simulink model "case1"  (R2024b)
settings: Solver=FixedStepAuto  StartTime=0  StopTime=1  FixedStep=1e-7  RelTol=1e-3
values from neighbouring files (symbols this model uses):
  SG_D_1_D = 0.01056    [IEEE9_case_parameters.m]    (also in case1_parameters.m; case2_parameters.m; case3_parameters.m; case4_parameters.m)
  SG_D_1_EnableSaturation = 0    [IEEE9_case_parameters.m]    (also in case1_parameters.m; case2_parameters.m; case3_parameters.m; case4_parameters.m)
  SG_D_1_f0 = 60    [IEEE9_case_parameters.m]    (also in case1_parameters.m; case2_parameters.m; case3_parameters.m; case4_parameters.m)
  SG_D_1_H = 7.5    [IEEE9_case_parameters.m]    (also in case1_parameters.m; case2_parameters.m; case3_parameters.m; case4_parameters.m)
  SG_D_1_K_A = 20    [IEEE9_case_parameters.m]    (also in case1_parameters.m; case2_parameters.m; case3_parameters.m; case4_parameters.m)
  SG_D_1_K_E = 1.000000e+1    (= 10)    [IEEE9_case_parameters.m]    (also in case1_parameters.m; case2_parameters.m; case3_parameters.m; case4_parameters.m)
  SG_D_1_K_F = 2.363    [IEEE9_case_parameters.m]    (also in case1_parameters.m; case2_parameters.m; case3_parameters.m; case4_parameters.m)
  SG_D_1_K_s = 0.5    [IEEE9_case_parameters.m]    (also in case1_parameters.m = 5; case2_parameters.m = 5; case3_parameters.m = 5; case4_parameters.m = 5)
  SG_D_1_R_a = 0.001088    [IEEE9_case_parameters.m]    (also in case1_parameters.m; case2_parameters.m; case3_parameters.m; case4_parameters.m)
  SG_D_1_S_A = 1    [IEEE9_case_parameters.m]    (also in case1_parameters.m; case2_parameters.m; case3_parameters.m; case4_parameters.m)
  SG_D_1_S_B = 0.103    [IEEE9_case_parameters.m]    (also in case1_parameters.m; case2_parameters.m; case3_parameters.m; case4_parameters.m)
  SG_D_1_S_N = 10.659857    [IEEE9_case_parameters.m]    (also in case1_parameters.m; case2_parameters.m; case3_parameters.m; case4_parameters.m)
  SG_D_1_SpeedPara = 200    [IEEE9_case_parameters.m]    (also in case1_parameters.m; case2_parameters.m; case3_parameters.m; case4_parameters.m)
  SG_D_1_T_0 = 0.720173    [IEEE9_case_parameters.m]    (also in case1_parameters.m = 0.755522; case2_parameters.m = 0.808931; case3_parameters.m = 0.869402; case4_parameters.m = 0.729316)
  SG_D_1_T_1 = 0.3    [IEEE9_case_parameters.m]    (also in case1_parameters.m; case2_parameters.m; case3_parameters.m; case4_parameters.m)
  SG_D_1_T_2 = 0.05    [IEEE9_case_parameters.m]    (also in case1_parameters.m; case2_parameters.m; case3_parameters.m; case4_parameters.m)
  SG_D_1_T_3 = 0.02    [IEEE9_case_parameters.m]    (also in case1_parameters.m; case2_parameters.m; case3_parameters.m; case4_parameters.m)
  SG_D_1_T_4 = 0.005    [IEEE9_case_parameters.m]    (also in case1_parameters.m; case2_parameters.m; case3_parameters.m; case4_parameters.m)
  SG_D_1_T_A = 0.02    [IEEE9_case_parameters.m]    (also in case1_parameters.m; case2_parameters.m; case3_parameters.m; case4_parameters.m)
  SG_D_1_T_dd = 8.000000e+0    (= 8)    [IEEE9_case_parameters.m]    (also in case1_parameters.m; case2_parameters.m; case3_parameters.m; case4_parameters.m)
  SG_D_1_T_ddd = 0.04    [IEEE9_case_parameters.m]    (also in case1_parameters.m; case2_parameters.m; case3_parameters.m; case4_parameters.m)
  SG_D_1_T_E = 0.314    [IEEE9_case_parameters.m]    (also in case1_parameters.m; case2_parameters.m; case3_parameters.m; case4_parameters.m)
  SG_D_1_T_F = 0.35    [IEEE9_case_parameters.m]    (also in case1_parameters.m; case2_parameters.m; case3_parameters.m; case4_parameters.m)
  SG_D_1_T_qd = 0.8    [IEEE9_case_parameters.m]    (also in case1_parameters.m; case2_parameters.m; case3_parameters.m; case4_parameters.m)
  SG_D_1_T_qdd = 0.02    [IEEE9_case_parameters.m]    (also in case1_parameters.m; case2_parameters.m; case3_parameters.m; case4_parameters.m)
  SG_D_1_T_speed = 0.1    [IEEE9_case_parameters.m]    (also in case1_parameters.m = 200; case2_parameters.m = 200; case3_parameters.m = 200; case4_parameters.m = 200)
  SG_D_1_T_w = 0.5    [IEEE9_case_parameters.m]    (also in case1_parameters.m; case2_parameters.m; case3_parameters.m; case4_parameters.m)
  SG_D_1_V_ref = 1.990276    [IEEE9_case_parameters.m]    (also in case1_parameters.m = 2.042296; case2_parameters.m = 2.051388; case3_parameters.m = 2.089584; case4_parameters.m = 2.01845)
  SG_D_1_w_ref = 376.991118    [IEEE9_case_parameters.m]    (also in case1_parameters.m; case2_parameters.m; case3_parameters.m; case4_parameters.m)
  SG_D_1_wb = 6.000000e+1    (= 60)    [IEEE9_case_parameters.m]    (also in case1_parameters.m; case2_parameters.m; case3_parameters.m; case4_parameters.m)
  SG_D_1_x_d = 1.9    [IEEE9_case_parameters.m]    (also in case1_parameters.m; case2_parameters.m; case3_parameters.m; case4_parameters.m)
  SG_D_1_x_dd = 0.302    [IEEE9_case_parameters.m]    (also in case1_parameters.m; case2_parameters.m; case3_parameters.m; case4_parameters.m)
  SG_D_1_x_ddd = 0.204    [IEEE9_case_parameters.m]    (also in case1_parameters.m; case2_parameters.m; case3_parameters.m; case4_parameters.m)
  SG_D_1_x_l = 0.05    [IEEE9_case_parameters.m]    (also in case1_parameters.m; case2_parameters.m; case3_parameters.m; case4_parameters.m)
  SG_D_1_x_q = 1.3    [IEEE9_case_parameters.m]    (also in case1_parameters.m; case2_parameters.m; case3_parameters.m; case4_parameters.m)
  SG_D_1_x_qd = 0.5    [IEEE9_case_parameters.m]    (also in case1_parameters.m; case2_parameters.m; case3_parameters.m; case4_parameters.m)
  SG_D_1_x_qdd = 0.3    [IEEE9_case_parameters.m]    (also in case1_parameters.m; case2_parameters.m; case3_parameters.m; case4_parameters.m)
  SG_D_2_D = 0.02    [IEEE9_case_parameters.m]    (also in case1_parameters.m; case2_parameters.m; case3_parameters.m; case4_parameters.m)
  SG_D_2_EnableSaturation = 0    [IEEE9_case_parameters.m]    (also in case1_parameters.m; case2_parameters.m; case3_parameters.m; case4_parameters.m)
  SG_D_2_f0 = 60    [IEEE9_case_parameters.m]    (also in case1_parameters.m; case2_parameters.m; case3_parameters.m; case4_parameters.m)
  SG_D_2_H = 8.000000e+0    (= 8)    [IEEE9_case_parameters.m]    (also in case1_parameters.m; case2_parameters.m; case3_parameters.m; case4_parameters.m)
  SG_D_2_K_A = 20    [IEEE9_case_parameters.m]    (also in case1_parameters.m; case2_parameters.m; case3_parameters.m; case4_parameters.m)
  SG_D_2_K_E = 1.000000e+1    (= 10)    [IEEE9_case_parameters.m]    (also in case1_parameters.m; case2_parameters.m; case3_parameters.m; case4_parameters.m)
  SG_D_2_K_F = 2.363    [IEEE9_case_parameters.m]    (also in case1_parameters.m; case2_parameters.m; case3_parameters.m; case4_parameters.m)
  SG_D_2_K_s = 0.5    [IEEE9_case_parameters.m]    (also in case1_parameters.m = 4; case2_parameters.m = 4; case3_parameters.m = 4; case4_parameters.m = 4)
  SG_D_2_R_a = 0.001088    [IEEE9_case_parameters.m]    (also in case1_parameters.m; case2_parameters.m; case3_parameters.m; case4_parameters.m)
  SG_D_2_S_A = 1    [IEEE9_case_parameters.m]    (also in case1_parameters.m; case2_parameters.m; case3_parameters.m; case4_parameters.m)
  SG_D_2_S_B = 0.103    [IEEE9_case_parameters.m]    (also in case1_parameters.m; case2_parameters.m; case3_parameters.m; case4_parameters.m)
  SG_D_2_S_N = 10.659857    [IEEE9_case_parameters.m]    (also in case1_parameters.m; case2_parameters.m; case3_parameters.m; case4_parameters.m)
  SG_D_2_SpeedPara = 200    [IEEE9_case_parameters.m]    (also in case1_parameters.m; case2_parameters.m; case3_parameters.m; case4_parameters.m)
  SG_D_2_T_0 = 1.632913    [IEEE9_case_parameters.m]    (also in case1_parameters.m = 1.632925; case2_parameters.m = 1.632915; case3_parameters.m = 1.632914; case4_parameters.m = 1.632927)
  SG_D_2_T_1 = 0.2    [IEEE9_case_parameters.m]    (also in case1_parameters.m; case2_parameters.m; case3_parameters.m; case4_parameters.m)
  SG_D_2_T_2 = 0.05    [IEEE9_case_parameters.m]    (also in case1_parameters.m; case2_parameters.m; case3_parameters.m; case4_parameters.m)
  SG_D_2_T_3 = 0.02    [IEEE9_case_parameters.m]    (also in case1_parameters.m; case2_parameters.m; case3_parameters.m; case4_parameters.m)
  SG_D_2_T_4 = 0.005    [IEEE9_case_parameters.m]    (also in case1_parameters.m; case2_parameters.m; case3_parameters.m; case4_parameters.m)
  SG_D_2_T_A = 0.02    [IEEE9_case_parameters.m]    (also in case1_parameters.m; case2_parameters.m; case3_parameters.m; case4_parameters.m)
  SG_D_2_T_dd = 7.9    [IEEE9_case_parameters.m]    (also in case1_parameters.m; case2_parameters.m; case3_parameters.m; case4_parameters.m)
  SG_D_2_T_ddd = 0.04    [IEEE9_case_parameters.m]    (also in case1_parameters.m; case2_parameters.m; case3_parameters.m; case4_parameters.m)
  SG_D_2_T_E = 0.314    [IEEE9_case_parameters.m]    (also in case1_parameters.m; case2_parameters.m; case3_parameters.m; case4_parameters.m)
  SG_D_2_T_F = 0.35    [IEEE9_case_parameters.m]    (also in case1_parameters.m; case2_parameters.m; case3_parameters.m; case4_parameters.m)
  SG_D_2_T_qd = 0.8    [IEEE9_case_parameters.m]    (also in case1_parameters.m; case2_parameters.m; case3_parameters.m; case4_parameters.m)
  SG_D_2_T_qdd = 0.015    [IEEE9_case_parameters.m]    (also in case1_parameters.m; case2_parameters.m; case3_parameters.m; case4_parameters.m)
  SG_D_2_T_speed = 0.1    [IEEE9_case_parameters.m]    (also in case1_parameters.m = 150; case2_parameters.m = 150; case3_parameters.m = 150; case4_parameters.m = 150)
  SG_D_2_T_w = 0.35    [IEEE9_case_parameters.m]    (also in case1_parameters.m; case2_parameters.m; case3_parameters.m; case4_parameters.m)
  SG_D_2_V_ref = 2.58547    [IEEE9_case_parameters.m]    (also in case1_parameters.m = 2.597896; case2_parameters.m = 2.587136; case3_parameters.m = 2.586042; case4_parameters.m = 2.599679)
  SG_D_2_w_ref = 376.991118    [IEEE9_case_parameters.m]    (also in case1_parameters.m; case2_parameters.m; case3_parameters.m; case4_parameters.m)
  SG_D_2_wb = 6.000000e+1    (= 60)    [IEEE9_case_parameters.m]    (also in case1_parameters.m; case2_parameters.m; case3_parameters.m; case4_parameters.m)
  SG_D_2_x_d = 1.8    [IEEE9_case_parameters.m]    (also in case1_parameters.m; case2_parameters.m; case3_parameters.m; case4_parameters.m)
  SG_D_2_x_dd = 0.302    [IEEE9_case_parameters.m]    (also in case1_parameters.m; case2_parameters.m; case3_parameters.m; case4_parameters.m)
  SG_D_2_x_ddd = 0.204    [IEEE9_case_parameters.m]    (also in case1_parameters.m; case2_parameters.m; case3_parameters.m; case4_parameters.m)
  SG_D_2_x_l = 0.05    [IEEE9_case_parameters.m]    (also in case1_parameters.m; case2_parameters.m; case3_parameters.m; case4_parameters.m)
  SG_D_2_x_q = 1.25    [IEEE9_case_parameters.m]    (also in case1_parameters.m; case2_parameters.m; case3_parameters.m; case4_parameters.m)
  SG_D_2_x_qd = 0.5    [IEEE9_case_parameters.m]    (also in case1_parameters.m; case2_parameters.m; case3_parameters.m; case4_parameters.m)
  SG_D_2_x_qdd = 0.3    [IEEE9_case_parameters.m]    (also in case1_parameters.m; case2_parameters.m; case3_parameters.m; case4_parameters.m)
  SG_D_3_D = 0.02    [IEEE9_case_parameters.m]    (also in case1_parameters.m; case2_parameters.m; case3_parameters.m; case4_parameters.m)
  SG_D_3_EnableSaturation = 0    [IEEE9_case_parameters.m]    (also in case1_parameters.m; case2_parameters.m; case3_parameters.m; case4_parameters.m)
  SG_D_3_f0 = 60    [IEEE9_case_parameters.m]    (also in case1_parameters.m; case2_parameters.m; case3_parameters.m; case4_parameters.m)
  SG_D_3_H = 7.7    [IEEE9_case_parameters.m]    (also in case1_parameters.m; case2_parameters.m; case3_parameters.m; case4_parameters.m)
  SG_D_3_K_A = 20    [IEEE9_case_parameters.m]    (also in case1_parameters.m; case2_parameters.m; case3_parameters.m; case4_parameters.m)
  SG_D_3_K_E = 1.000000e+1    (= 10)    [IEEE9_case_parameters.m]    (also in case1_parameters.m; case2_parameters.m; case3_parameters.m; case4_parameters.m)
  SG_D_3_K_F = 2.363    [IEEE9_case_parameters.m]    (also in case1_parameters.m; case2_parameters.m; case3_parameters.m; case4_parameters.m)
  SG_D_3_K_s = 0.2    [IEEE9_case_parameters.m]    (also in case1_parameters.m = 2; case2_parameters.m = 2; case3_parameters.m = 2; case4_parameters.m = 2)
  SG_D_3_R_a = 0.001088    [IEEE9_case_parameters.m]    (also in case1_parameters.m; case2_parameters.m; case3_parameters.m; case4_parameters.m)
  SG_D_3_S_A = 1    [IEEE9_case_parameters.m]    (also in case1_parameters.m; case2_parameters.m; case3_parameters.m; case4_parameters.m)
  SG_D_3_S_B = 0.103    [IEEE9_case_parameters.m]    (also in case1_parameters.m; case2_parameters.m; case3_parameters.m; case4_parameters.m)
  SG_D_3_S_N = 10.659857    [IEEE9_case_parameters.m]    (also in case1_parameters.m; case2_parameters.m; case3_parameters.m; case4_parameters.m)
  SG_D_3_SpeedPara = 200    [IEEE9_case_parameters.m]    (also in case1_parameters.m; case2_parameters.m; case3_parameters.m; case4_parameters.m)
  SG_D_3_T_0 = 0.850788    [IEEE9_case_parameters.m]    (also in case1_parameters.m = 0.850786; case2_parameters.m = 0.850787; case3_parameters.m; case4_parameters.m = 0.850786)
  SG_D_3_T_1 = 0.2    [IEEE9_case_parameters.m]    (also in case1_parameters.m; case2_parameters.m; case3_parameters.m; case4_parameters.m)
  SG_D_3_T_2 = 0.05    [IEEE9_case_parameters.m]    (also in case1_parameters.m; case2_parameters.m; case3_parameters.m; case4_parameters.m)
  SG_D_3_T_3 = 0.02    [IEEE9_case_parameters.m]    (also in case1_parameters.m; case2_parameters.m; case3_parameters.m; case4_parameters.m)
  SG_D_3_T_4 = 0.005    [IEEE9_case_parameters.m]    (also in case1_parameters.m; case2_parameters.m; case3_parameters.m; case4_parameters.m)
  SG_D_3_T_A = 0.02    [IEEE9_case_parameters.m]    (also in case1_parameters.m; case2_parameters.m; case3_parameters.m; case4_parameters.m)
  SG_D_3_T_dd = 8.1    [IEEE9_case_parameters.m]    (also in case1_parameters.m; case2_parameters.m; case3_parameters.m; case4_parameters.m)
  SG_D_3_T_ddd = 0.04    [IEEE9_case_parameters.m]    (also in case1_parameters.m; case2_parameters.m; case3_parameters.m; case4_parameters.m)
  SG_D_3_T_E = 0.314    [IEEE9_case_parameters.m]    (also in case1_parameters.m; case2_parameters.m; case3_parameters.m; case4_parameters.m)
  SG_D_3_T_F = 0.35    [IEEE9_case_parameters.m]    (also in case1_parameters.m; case2_parameters.m; case3_parameters.m; case4_parameters.m)
  SG_D_3_T_qd = 0.8    [IEEE9_case_parameters.m]    (also in case1_parameters.m; case2_parameters.m; case3_parameters.m; case4_parameters.m)
  SG_D_3_T_qdd = 0.015    [IEEE9_case_parameters.m]    (also in case1_parameters.m; case2_parameters.m; case3_parameters.m; case4_parameters.m)
  SG_D_3_T_speed = 0.1    [IEEE9_case_parameters.m]    (also in case1_parameters.m = 180; case2_parameters.m = 180; case3_parameters.m = 180; case4_parameters.m = 180)
  SG_D_3_T_w = 0.4    [IEEE9_case_parameters.m]    (also in case1_parameters.m; case2_parameters.m; case3_parameters.m; case4_parameters.m)
  SG_D_3_V_ref = 1.892727    [IEEE9_case_parameters.m]    (also in case1_parameters.m = 1.906439; case2_parameters.m = 1.895535; case3_parameters.m = 1.892105; case4_parameters.m = 1.906598)
  SG_D_3_w_ref = 376.991118    [IEEE9_case_parameters.m]    (also in case1_parameters.m; case2_parameters.m; case3_parameters.m; case4_parameters.m)
  SG_D_3_wb = 6.000000e+1    (= 60)    [IEEE9_case_parameters.m]    (also in case1_parameters.m; case2_parameters.m; case3_parameters.m; case4_parameters.m)
  SG_D_3_x_d = 1.85    [IEEE9_case_parameters.m]    (also in case1_parameters.m; case2_parameters.m; case3_parameters.m; case4_parameters.m)
  SG_D_3_x_dd = 0.302    [IEEE9_case_parameters.m]    (also in case1_parameters.m; case2_parameters.m; case3_parameters.m; case4_parameters.m)
  SG_D_3_x_ddd = 0.204    [IEEE9_case_parameters.m]    (also in case1_parameters.m; case2_parameters.m; case3_parameters.m; case4_parameters.m)
  SG_D_3_x_l = 0.05    [IEEE9_case_parameters.m]    (also in case1_parameters.m; case2_parameters.m; case3_parameters.m; case4_parameters.m)
  SG_D_3_x_q = 1.2    [IEEE9_case_parameters.m]    (also in case1_parameters.m; case2_parameters.m; case3_parameters.m; case4_parameters.m)
  SG_D_3_x_qd = 0.5    [IEEE9_case_parameters.m]    (also in case1_parameters.m; case2_parameters.m; case3_parameters.m; case4_parameters.m)
  SG_D_3_x_qdd = 0.3    [IEEE9_case_parameters.m]    (also in case1_parameters.m; case2_parameters.m; case3_parameters.m; case4_parameters.m)
(part 8 of 12)

== system case1/SG_D_2/d_psi_d_SG_D_2_block ==
  note: d_psi_d_SG_D_2 in case1
      | $2\,\pi \,f_{0}\,\left(v_{d,\mathrm{SG},D,2}\,\sin\left(\theta _{\mathrm{SG},D,2}\right)-v_{q,\mathrm{SG},D,2}\,\cos\left(\theta _{\mathrm{SG},D,2}\right)+\frac{R_{a}\,\left(\frac{\psi _{\mathrm{1d},\mathrm{SG},D,2}\,\left(x_{\mathrm{dd}}-x_{\mathrm{ddd}}\right)}{x_{\mathrm{dd}}-x_{l}}-\psi _{d,\mathrm{SG},D,2}+\frac{\psi _{\mathrm{fd},\mathrm{SG},D,2}\,\left(x_{\mathrm{ddd}}-x_{l}\right)}{x_{\mathrm{dd}}-x_{l}}\right)}{x_{\mathrm{ddd}}}+\frac{\psi _{q,\mathrm{SG},D,2}\,w_{\mathrm{SG},D,2}}{2\,f_{0}\,\pi }\right)$
      | Automatically generated on 2025-10-31 18:48:10 .
  State_psi_1d_SG_D_2_48ea4 : Inport
  State_psi_d_SG_D_2_8d25d : Inport  Port=2
  State_psi_fd_SG_D_2_4d493 : Inport  Port=3
  Input_v_d_SG_D_2_e74d4 : Inport  Port=4
  State_theta_SG_D_2_cb884 : Inport  Port=5
  Input_v_q_SG_D_2_ef7b1 : Inport  Port=6
  State_theta_SG_D_2_069cc : Inport  Port=7
  State_psi_q_SG_D_2_06491 : Inport  Port=8
  State_w_SG_D_2_46e5d : Inport  Port=9
  Add_9594a : Sum
  Add_a58f5 : Sum
  Constant_-1_bbc80 : Constant  Value=-1
  Constant_-2.0_5abee : Constant  Value=-2.0
  Constant_2.0_c2643 : Constant  Value=2.0
  Constant_R_a_77be8 : Constant  Value=R_a
  Constant_f0_ecad6 : Constant  Value=f0
  Constant_f0_ecc70 : Constant  Value=f0
  Constant_pi_1b2b5 : Constant  Value=pi
  Constant_pi_ab6a4 : Constant  Value=pi
  Constant_x_dd_4634c : Constant  Value=x_dd
  Constant_x_dd_53177 : Constant  Value=x_dd
  Constant_x_dd_7f193 : Constant  Value=x_dd
  Constant_x_ddd_27663 : Constant  Value=x_ddd
  Constant_x_ddd_2f050 : Constant  Value=x_ddd
  Constant_x_ddd_407bb : Constant  Value=x_ddd
  Constant_x_l_0d10b : Constant  Value=x_l
  Constant_x_l_b133c : Constant  Value=x_l
  Constant_x_l_d501e : Constant  Value=x_l
  Divide_2553b : Product  Inputs=*/
  Divide_6fe8b : Product  Inputs=*/
  Divide_88a68 : Product  Inputs=*/
  Divide_89ce0 : Product  Inputs=*/
  MathFunc_cos_0fde2 : Trigonometry  Operator=cos
  MathFunc_sin_788f3 : Trigonometry
  Product_269c7 : Product
  Product_5eb09 : Product
  Product_94f92 : Product
  Product_9e7bd : Product
  Product_a0a07 : Product
  Product_b26e1 : Product
  Product_d5dea : Product
  Product_d6782 : Product
  Product_ea208 : Product
  Product_eca76 : Product
  Product_f9e18 : Product
  Product_fe3b7 : Product
  Subtract_6ad03 : Sum  Inputs=+-
  Subtract_6defb : Sum  Inputs=+-
  Subtract_826d9 : Sum  Inputs=+-
  Subtract_837ee : Sum  Inputs=+-
  Subtract_881d5 : Sum  Inputs=+-
  Subtract_8d79c : Sum  Inputs=+-
  Subtract_f6c5f : Sum  Inputs=+-
  Blockout_d_psi_d_SG_D_2_591f5 : Outport
  wires:
  MathFunc_sin_788f3/1 -> Product_f9e18/2
  Constant_x_dd_53177/1 -> Subtract_826d9/1
  Constant_-1_bbc80/1 -> Product_eca76/1
  Constant_x_l_d501e/1 -> Subtract_826d9/2
  State_psi_1d_SG_D_2_48ea4/1 -> Product_eca76/2
  Constant_f0_ecad6/1 -> Product_ea208/2
  Constant_2.0_c2643/1 -> Product_94f92/1
  Constant_x_l_0d10b/1 -> Subtract_881d5/2
  Constant_x_dd_7f193/1 -> Subtract_6ad03/1
  Product_d5dea/1 -> Blockout_d_psi_d_SG_D_2_591f5/1
  Constant_pi_1b2b5/1 -> Product_94f92/2
  Constant_x_ddd_407bb/1 -> Subtract_6ad03/2
  Subtract_f6c5f/1 -> Product_d5dea/2
  Product_eca76/1 -> Product_fe3b7/1
  Product_94f92/1 -> Product_d6782/1
  Subtract_6ad03/1 -> Product_fe3b7/2
  Divide_89ce0/1 -> Subtract_f6c5f/2
  Constant_x_ddd_27663/1 -> Subtract_6defb/1
  Constant_x_l_b133c/1 -> Subtract_6defb/2
  Product_fe3b7/1 -> Divide_6fe8b/1
  Subtract_8d79c/1 -> Add_9594a/1
  Subtract_826d9/1 -> Divide_6fe8b/2
  State_psi_fd_SG_D_2_4d493/1 -> Product_9e7bd/1
  Subtract_6defb/1 -> Product_9e7bd/2
  Constant_x_dd_4634c/1 -> Subtract_881d5/1
  Divide_6fe8b/1 -> Add_a58f5/1
  State_psi_d_SG_D_2_8d25d/1 -> Add_a58f5/2
  Product_9e7bd/1 -> Divide_2553b/1
  Subtract_881d5/1 -> Divide_2553b/2
  Add_a58f5/1 -> Subtract_837ee/1
  Divide_2553b/1 -> Subtract_837ee/2
  Constant_R_a_77be8/1 -> Product_b26e1/1
  Subtract_837ee/1 -> Product_b26e1/2
  Divide_88a68/1 -> Subtract_8d79c/1
  State_theta_SG_D_2_cb884/1 -> MathFunc_sin_788f3/1
  Product_b26e1/1 -> Divide_88a68/1
  Constant_-2.0_5abee/1 -> Product_a0a07/1
  Input_v_d_SG_D_2_e74d4/1 -> Product_f9e18/1
  Constant_x_ddd_2f050/1 -> Divide_88a68/2
  State_theta_SG_D_2_069cc/1 -> MathFunc_cos_0fde2/1
  Product_ea208/1 -> Product_d5dea/1
  Product_f9e18/1 -> Subtract_8d79c/2
  Product_a0a07/1 -> Product_ea208/1
  Input_v_q_SG_D_2_ef7b1/1 -> Product_269c7/1
  MathFunc_cos_0fde2/1 -> Product_269c7/2
  State_psi_q_SG_D_2_06491/1 -> Product_5eb09/1
  State_w_SG_D_2_46e5d/1 -> Product_5eb09/2
  Constant_f0_ecc70/1 -> Product_d6782/2
  Constant_pi_ab6a4/1 -> Product_a0a07/2
  Product_269c7/1 -> Add_9594a/2
  Product_5eb09/1 -> Divide_89ce0/1
  Product_d6782/1 -> Divide_89ce0/2
  Add_9594a/1 -> Subtract_f6c5f/1

== system case1/SG_D_2/d_psi_fd_SG_D_2_block ==
  note: d_psi_fd_SG_D_2 in case1
      | $-\frac{\psi _{\mathrm{fd},\mathrm{SG},D,2}-E_{\mathrm{fd},\mathrm{SG},D,2}+\left(x_{d}-x_{\mathrm{dd}}\right)\,\left(\frac{\frac{\psi _{\mathrm{1d},\mathrm{SG},D,2}\,\left(x_{\mathrm{dd}}-x_{\mathrm{ddd}}\right)}{x_{\mathrm{dd}}-x_{l}}-\psi _{d,\mathrm{SG},D,2}+\frac{\psi _{\mathrm{fd},\mathrm{SG},D,2}\,\left(x_{\mathrm{ddd}}-x_{l}\right)}{x_{\mathrm{dd}}-x_{l}}}{x_{\mathrm{ddd}}}-\frac{\left(x_{\mathrm{dd}}-x_{\mathrm{ddd}}\right)\,\left(\psi _{\mathrm{1d},\mathrm{SG},D,2}-\psi _{\mathrm{fd},\mathrm{SG},D,2}+\frac{\left(x_{\mathrm{dd}}-x_{l}\right)\,\left(\frac{\psi _{\mathrm{1d},\mathrm{SG},D,2}\,\left(x_{\mathrm{dd}}-x_{\mathrm{ddd}}\right)}{x_{\mathrm{dd}}-x_{l}}-\psi _{d,\mathrm{SG},D,2}+\frac{\psi _{\mathrm{fd},\mathrm{SG},D,2}\,\left(x_{\mathrm{ddd}}-x_{l}\right)}{x_{\mathrm{dd}}-x_{l}}\right)}{x_{\mathrm{ddd}}}\right)}{{\left(x_{\mathrm{dd}}-x_{l}\right)}^2}\right)}{T_{\mathrm{dd}}}$
      | Automatically generated on 2025-10-31 18:48:19 .
  State_E_fd_SG_D_2_9c9d0 : Inport
  State_psi_fd_SG_D_2_87c43 : Inport  Port=2
  State_psi_1d_SG_D_2_cf418 : Inport  Port=3
  State_psi_fd_SG_D_2_c572b : Inport  Port=4
  State_psi_1d_SG_D_2_6822c : Inport  Port=5
  State_psi_d_SG_D_2_85721 : Inport  Port=6
  State_psi_fd_SG_D_2_150ec : Inport  Port=7
  State_psi_1d_SG_D_2_241cc : Inport  Port=8
  State_psi_d_SG_D_2_887e8 : Inport  Port=9
  State_psi_fd_SG_D_2_9d902 : Inport  Port=10
  Add_517b2 : Sum
  Add_9a366 : Sum
  Constant_-1_266e8 : Constant  Value=-1
  Constant_-1_7de64 : Constant  Value=-1
  Constant_-1_ecdc1 : Constant  Value=-1
  Constant_2.0_2a87b : Constant  Value=2.0
  Constant_T_dd_17eae : Constant  Value=T_dd
  Constant_x_d_af99e : Constant  Value=x_d
  Constant_x_dd_078d5 : Constant  Value=x_dd
  Constant_x_dd_2af89 : Constant  Value=x_dd
  Constant_x_dd_5ad05 : Constant  Value=x_dd
  Constant_x_dd_62f78 : Constant  Value=x_dd
  Constant_x_dd_70df7 : Constant  Value=x_dd
  Constant_x_dd_86249 : Constant  Value=x_dd
  Constant_x_dd_cf584 : Constant  Value=x_dd
  Constant_x_dd_f24ca : Constant  Value=x_dd
  Constant_x_dd_f6118 : Constant  Value=x_dd
  Constant_x_dd_fa9c5 : Constant  Value=x_dd
  Constant_x_ddd_246be : Constant  Value=x_ddd
  Constant_x_ddd_5c82d : Constant  Value=x_ddd
  Constant_x_ddd_87f9c : Constant  Value=x_ddd
  Constant_x_ddd_88a27 : Constant  Value=x_ddd
  Constant_x_ddd_b6581 : Constant  Value=x_ddd
  Constant_x_ddd_ea990 : Constant  Value=x_ddd
  Constant_x_ddd_eb8c0 : Constant  Value=x_ddd
  Constant_x_l_35564 : Constant  Value=x_l
  Constant_x_l_50fda : Constant  Value=x_l
  Constant_x_l_54d6d : Constant  Value=x_l
  Constant_x_l_5e86d : Constant  Value=x_l
  Constant_x_l_9cb25 : Constant  Value=x_l
  Constant_x_l_c80b3 : Constant  Value=x_l
  Constant_x_l_d4bdf : Constant  Value=x_l
  Constant_x_l_dd037 : Constant  Value=x_l
  Divide_50a2c : Product  Inputs=*/
  Divide_5573a : Product  Inputs=*/
  Divide_5d351 : Product  Inputs=*/
  Divide_8425e : Product  Inputs=*/
  Divide_8de76 : Product  Inputs=*/
  Divide_a9e35 : Product  Inputs=*/
  Divide_b94e7 : Product  Inputs=*/
  Divide_e9fad : Product  Inputs=*/
  Power_e99dd : Math  Operator=pow
  Product_0ff69 : Product
  Product_1c511 : Product
  Product_28470 : Product
  Product_373a0 : Product
  Product_7702b : Product
  Product_9044e : Product
  Product_b1fa7 : Product
  Product_f2e05 : Product
  Product_fc601 : Product
  Product_fe086 : Product
  Subtract_15082 : Sum  Inputs=+-
  Subtract_154bb : Sum  Inputs=+-
  Subtract_35d70 : Sum  Inputs=+-
  Subtract_3df41 : Sum  Inputs=+-
  Subtract_41d15 : Sum  Inputs=+-
  Subtract_423ac : Sum  Inputs=+-
  Subtract_66846 : Sum  Inputs=+-
  Subtract_8565d : Sum  Inputs=+-
  Subtract_a164d : Sum  Inputs=+-
  Subtract_a41c0 : Sum  Inputs=+-
  Subtract_cb11c : Sum  Inputs=+-
  Subtract_cf430 : Sum  Inputs=+-
  Subtract_d96e7 : Sum  Inputs=+-
  Subtract_ec12e : Sum  Inputs=+-
  Subtract_f1009 : Sum  Inputs=+-
  Subtract_f3e93 : Sum  Inputs=+-
  Subtract_f8fbb : Sum  Inputs=+-
  Subtract_f98c3 : Sum  Inputs=+-
  Subtract_fe805 : Sum  Inputs=+-
  Blockout_d_psi_fd_SG_D_2_b0c7a : Outport
  wires:
  Constant_x_dd_fa9c5/1 -> Subtract_15082/1
  Constant_-1_ecdc1/1 -> Product_1c511/1
  Constant_x_l_d4bdf/1 -> Subtract_f3e93/2
  Divide_5d351/1 -> Add_517b2/1
  Subtract_f8fbb/1 -> Product_f2e05/2
  Constant_x_l_c80b3/1 -> Subtract_15082/2
  Product_f2e05/1 -> Divide_8de76/1
  State_psi_1d_SG_D_2_6822c/1 -> Product_1c511/2
  Constant_x_dd_86249/1 -> Subtract_8565d/1
  Product_9044e/1 -> Divide_5d351/1
  Constant_x_dd_f6118/1 -> Subtract_fe805/1
  Constant_x_ddd_87f9c/1 -> Subtract_8565d/2
  Constant_x_dd_2af89/1 -> Subtract_f1009/1
  Product_1c511/1 -> Product_7702b/1
  Subtract_8565d/1 -> Product_7702b/2
  State_psi_d_SG_D_2_887e8/1 -> Add_517b2/2
  Constant_x_ddd_246be/1 -> Subtract_f8fbb/1
  Constant_x_l_dd037/1 -> Subtract_f8fbb/2
  Product_7702b/1 -> Divide_8425e/1
  Subtract_15082/1 -> Divide_8425e/2
  State_psi_fd_SG_D_2_150ec/1 -> Product_f2e05/1
  Subtract_35d70/1 -> Product_0ff69/2
  Constant_x_dd_62f78/1 -> Subtract_a164d/1
  Constant_x_l_35564/1 -> Subtract_a164d/2
  Product_28470/1 -> Product_0ff69/1
  Divide_8425e/1 -> Add_9a366/1
  State_psi_d_SG_D_2_85721/1 -> Add_9a366/2
  Subtract_a164d/1 -> Divide_8de76/2
  Constant_x_dd_cf584/1 -> Subtract_f3e93/1
  Constant_x_ddd_88a27/1 -> Subtract_ec12e/1
  Add_9a366/1 -> Subtract_66846/1
  Divide_8de76/1 -> Subtract_66846/2
  Constant_-1_266e8/1 -> Product_373a0/1
  Product_fc601/1 -> Divide_50a2c/1
  State_psi_1d_SG_D_2_241cc/1 -> Product_373a0/2
  Subtract_fe805/1 -> Product_28470/2
  Constant_x_dd_f24ca/1 -> Subtract_3df41/1
  Divide_50a2c/1 -> Subtract_cb11c/2
  Constant_-1_7de64/1 -> Product_28470/1
  Constant_x_ddd_b6581/1 -> Subtract_3df41/2
  Constant_x_ddd_5c82d/1 -> Divide_b94e7/2
  Subtract_f3e93/1 -> Product_fe086/1
  Subtract_66846/1 -> Product_fe086/2
  State_psi_fd_SG_D_2_c572b/1 -> Subtract_41d15/2
  Product_373a0/1 -> Product_9044e/1
  Subtract_3df41/1 -> Product_9044e/2
  Constant_2.0_2a87b/1 -> Power_e99dd/2
  State_psi_1d_SG_D_2_cf418/1 -> Subtract_41d15/1
  Constant_x_dd_5ad05/1 -> Subtract_154bb/1
  Subtract_ec12e/1 -> Product_fc601/2
  Constant_x_l_5e86d/1 -> Subtract_154bb/2
  Constant_x_l_9cb25/1 -> Subtract_ec12e/2
  Constant_x_ddd_ea990/1 -> Subtract_fe805/2
  Subtract_f1009/1 -> Divide_50a2c/2
  Product_fe086/1 -> Divide_b94e7/1
  Subtract_154bb/1 -> Divide_5d351/2
  State_psi_fd_SG_D_2_9d902/1 -> Product_fc601/1
  Constant_x_l_50fda/1 -> Subtract_f1009/2
  Constant_x_dd_70df7/1 -> Subtract_cf430/1
  Subtract_41d15/1 -> Subtract_35d70/1
  Divide_b94e7/1 -> Subtract_35d70/2
  Constant_x_l_54d6d/1 -> Subtract_cf430/2
  Subtract_cf430/1 -> Power_e99dd/1
  Add_517b2/1 -> Subtract_cb11c/1
  Product_0ff69/1 -> Divide_e9fad/1
  Power_e99dd/1 -> Divide_e9fad/2
  Subtract_cb11c/1 -> Divide_5573a/1
  Constant_x_ddd_eb8c0/1 -> Divide_5573a/2
  Constant_x_d_af99e/1 -> Subtract_f98c3/1
  Constant_x_dd_078d5/1 -> Subtract_f98c3/2
  Divide_e9fad/1 -> Subtract_d96e7/1
  Divide_5573a/1 -> Subtract_d96e7/2
  State_E_fd_SG_D_2_9c9d0/1 -> Subtract_423ac/1
  State_psi_fd_SG_D_2_87c43/1 -> Subtract_423ac/2
  Subtract_f98c3/1 -> Product_b1fa7/1
  Subtract_d96e7/1 -> Product_b1fa7/2
  Subtract_423ac/1 -> Subtract_a41c0/1
  Product_b1fa7/1 -> Subtract_a41c0/2
  Subtract_a41c0/1 -> Divide_a9e35/1
  Constant_T_dd_17eae/1 -> Divide_a9e35/2
  Divide_a9e35/1 -> Blockout_d_psi_fd_SG_D_2_b0c7a/1

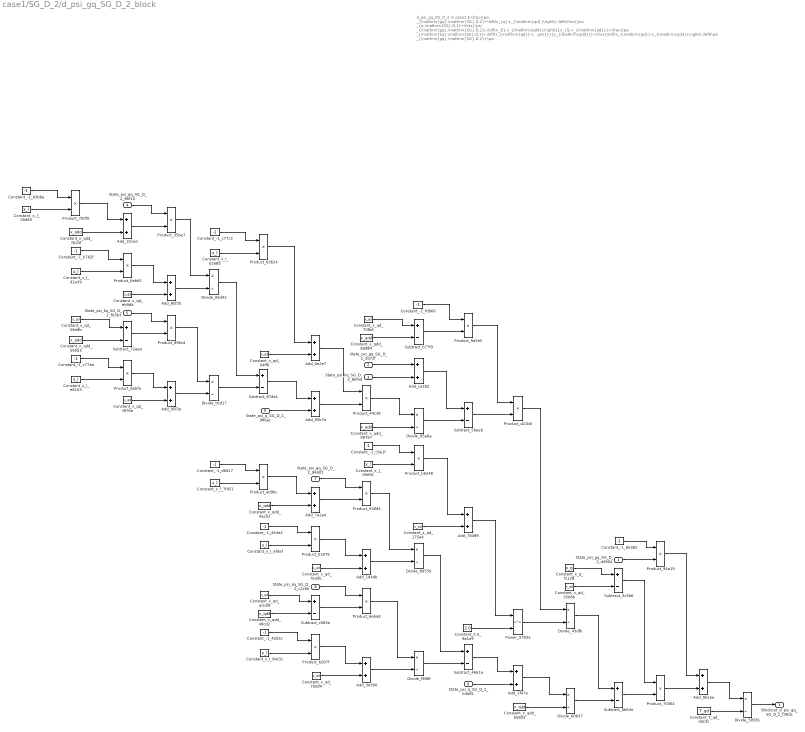
== system case1/SG_D_2/d_psi_gq_SG_D_2_block ==
  note: d_psi_gq_SG_D_2 in case1
      | $-\frac{\psi _{\mathrm{gq},\mathrm{SG},D,2}+\left(x_{q}-x_{\mathrm{qd}}\right)\,\left(\frac{\psi _{q,\mathrm{SG},D,2}+\frac{\psi _{\mathrm{gq},\mathrm{SG},D,2}\,\left(x_{l}-x_{\mathrm{qdd}}\right)}{x_{l}-x_{\mathrm{qd}}}+\frac{\psi _{\mathrm{kq},\mathrm{SG},D,2}\,\left(x_{\mathrm{qd}}-x_{\mathrm{qdd}}\right)}{x_{l}-x_{\mathrm{qd}}}}{x_{\mathrm{qdd}}}+\frac{\left(x_{\mathrm{qd}}-x_{\mathrm{qdd}}\right)\,\left(\psi _{\mathrm{gq},\mathrm{SG},D,2}+\psi _{\mathrm{kq},\mathrm{SG},D,2}+\frac{\left(x_{l}-x_{\mathrm{qd}}\right)\,\left(\psi _{q,\mathrm{SG},D,2}+\frac{\psi _{\mathrm{gq},\mathrm{SG},D,2}\,\left(x_{l}-x_{\mathrm{qdd}}\right)}{x_{l}-x_{\mathrm{qd}}}+\frac{\psi _{\mathrm{kq},\mathrm{SG},D,2}\,\left(x_{\mathrm{qd}}-x_{\mathrm{qdd}}\right)}{x_{l}-x_{\mathrm{qd}}}\right)}{x_{\mathrm{qdd}}}\right)}{{\left(x_{l}-x_{\mathrm{qd}}\right)}^2}\right)}{T_{\mathrm{qd}}}$
      | Automatically generated on 2025-10-31 18:48:28 .
  State_psi_gq_SG_D_2_d4904 : Inport
  State_psi_gq_SG_D_2_2d72f : Inport  Port=2
  State_psi_kq_SG_D_2_8efed : Inport  Port=3
  State_psi_gq_SG_D_2_96f10 : Inport  Port=4
  State_psi_kq_SG_D_2_f03b3 : Inport  Port=5
  State_psi_q_SG_D_2_986ec : Inport  Port=6
  State_psi_gq_SG_D_2_84d01 : Inport  Port=7
  State_psi_kq_SG_D_2_c2c6b : Inport  Port=8
  State_psi_q_SG_D_2_b4e81 : Inport  Port=9
  Add_1d4db : Sum
  Add_1f47e : Sum
  Add_32ced : Sum
  Add_3d300 : Sum
  Add_6e2e7 : Sum
  Add_78499 : Sum
  Add_7a2a4 : Sum
  Add_80f35 : Sum
  Add_95b7a : Sum
  Add_95f2e : Sum
  Add_9b1ee : Sum
  Add_ca182 : Sum
  Constant_-1_42b5c : Constant  Value=-1
  Constant_-1_464e4 : Constant  Value=-1
  Constant_-1_6b382 : Constant  Value=-1
  Constant_-1_b3b6a : Constant  Value=-1
  Constant_-1_b762f : Constant  Value=-1
  Constant_-1_c77aa : Constant  Value=-1
  Constant_-1_c77c3 : Constant  Value=-1
  Constant_-1_c9a1f : Constant  Value=-1
  Constant_-1_d6d17 : Constant  Value=-1
  Constant_-1_fd960 : Constant  Value=-1
  Constant_2.0_9a1e9 : Constant  Value=2.0
  Constant_T_qd_ddc3c : Constant  Value=T_qd
  Constant_x_l_00d83 : Constant  Value=x_l
  Constant_x_l_02685 : Constant  Value=x_l
  Constant_x_l_09e91 : Constant  Value=x_l
  Constant_x_l_7f451 : Constant  Value=x_l
  Constant_x_l_84c5c : Constant  Value=x_l
  Constant_x_l_d2a39 : Constant  Value=x_l
  Constant_x_l_e6103 : Constant  Value=x_l
  Constant_x_l_efdef : Constant  Value=x_l
  Constant_x_q_fc128 : Constant  Value=x_q
  Constant_x_qd_04ff6 : Constant  Value=x_qd
  Constant_x_qd_175a4 : Constant  Value=x_qd
  Constant_x_qd_3568b : Constant  Value=x_qd
  Constant_x_qd_56e8b : Constant  Value=x_qd
  Constant_x_qd_70504 : Constant  Value=x_qd
  Constant_x_qd_70fb6 : Constant  Value=x_qd
  Constant_x_qd_acb58 : Constant  Value=x_qd
  Constant_x_qd_eb9db : Constant  Value=x_qd
  Constant_x_qd_f876e : Constant  Value=x_qd
  Constant_x_qd_fe35b : Constant  Value=x_qd
  Constant_x_qdd_48cd2 : Constant  Value=x_qdd
  Constant_x_qdd_4acd1 : Constant  Value=x_qdd
  Constant_x_qdd_590a3 : Constant  Value=x_qdd
  Constant_x_qdd_7b24f : Constant  Value=x_qdd
  Constant_x_qdd_8d984 : Constant  Value=x_qdd
  Constant_x_qdd_98767 : Constant  Value=x_qdd
  Constant_x_qdd_b5603 : Constant  Value=x_qdd
  Divide_06d42 : Product  Inputs=*/
  Divide_43dfb : Product  Inputs=*/
  Divide_58581 : Product  Inputs=*/
  Divide_60637 : Product  Inputs=*/
  Divide_85a6a : Product  Inputs=*/
  Divide_8d550 : Product  Inputs=*/
  Divide_dcd17 : Product  Inputs=*/
  Divide_f898f : Product  Inputs=*/
  Power_5783a : Math  Operator=pow
  Product_01876 : Product
  Product_0eb65 : Product
  Product_35be7 : Product
  Product_44c38 : Product
  Product_6abfe : Product
  Product_6eba8 : Product
  Product_70064 : Product
  Product_700f0 : Product
  Product_896cd : Product
  Product_938d5 : Product
  Product_94a19 : Product
  Product_9a5e5 : Product
  Product_a09bc : Product
  Product_b207f : Product
  Product_b3b24 : Product
  Product_b6248 : Product
  Product_d21b6 : Product
  Subtract_3c5b6 : Sum  Inputs=+-
  Subtract_4661a : Sum  Inputs=+-
  Subtract_56eeb : Sum  Inputs=+-
  Subtract_6b63e : Sum  Inputs=+-
  Subtract_72aee : Sum  Inputs=+-
  Subtract_87da1 : Sum  Inputs=+-
  Subtract_b77f9 : Sum  Inputs=+-
  Subtract_c083a : Sum  Inputs=+-
  Blockout_d_psi_gq_SG_D_2_f38dc : Outport
  wires:
  Constant_x_l_84c5c/1 -> Product_b207f/2
  Constant_x_l_7f451/1 -> Product_a09bc/2
  Constant_x_qd_56e8b/1 -> Subtract_72aee/1
  Constant_x_l_09e91/1 -> Product_b6248/2
  Constant_x_qdd_8d984/1 -> Subtract_b77f9/2
  Constant_-1_c77aa/1 -> Product_6abfe/1
  Constant_-1_b3b6a/1 -> Product_700f0/1
  State_psi_gq_SG_D_2_2d72f/1 -> Add_ca182/1
  Constant_x_qdd_590a3/1 -> Subtract_72aee/2
  Constant_x_qd_70fb6/1 -> Subtract_b77f9/1
  Constant_x_l_e6103/1 -> Product_6abfe/2
  Constant_x_l_00d83/1 -> Product_700f0/2
  Product_6abfe/1 -> Add_95f2e/1
  Product_700f0/1 -> Add_32ced/1
  Constant_x_l_d2a39/1 -> Product_0eb65/2
  Constant_x_l_02685/1 -> Product_b3b24/2
  Constant_x_qd_f876e/1 -> Add_95f2e/2
  Constant_x_qdd_7b24f/1 -> Add_32ced/2
  Constant_-1_b762f/1 -> Product_0eb65/1
  Constant_x_qd_70504/1 -> Add_3d300/2
  Constant_x_qdd_4acd1/1 -> Add_7a2a4/2
  State_psi_gq_SG_D_2_96f10/1 -> Product_35be7/1
  Add_95f2e/1 -> Divide_dcd17/2
  Add_32ced/1 -> Product_35be7/2
  Constant_x_qd_3568b/1 -> Subtract_3c5b6/2
  Product_0eb65/1 -> Add_80f35/1
  Constant_x_qd_eb9db/1 -> Add_80f35/2
  State_psi_kq_SG_D_2_f03b3/1 -> Product_896cd/1
  Divide_06d42/1 -> Subtract_87da1/1
  Subtract_72aee/1 -> Product_896cd/2
  Product_35be7/1 -> Divide_06d42/1
  Add_80f35/1 -> Divide_06d42/2
  Add_95b7a/1 -> Product_44c38/2
  Product_896cd/1 -> Divide_dcd17/1
  Constant_-1_c77c3/1 -> Product_b3b24/1
  Divide_dcd17/1 -> Subtract_87da1/2
  Constant_-1_42b5c/1 -> Product_b207f/1
  Constant_-1_d6d17/1 -> Product_a09bc/1
  Product_b3b24/1 -> Add_6e2e7/1
  Constant_x_qdd_48cd2/1 -> Subtract_c083a/2
  Constant_x_qd_04ff6/1 -> Add_6e2e7/2
  Subtract_87da1/1 -> Add_95b7a/1
  Constant_-1_c9a1f/1 -> Product_b6248/1
  State_psi_q_SG_D_2_986ec/1 -> Add_95b7a/2
  Product_b207f/1 -> Add_3d300/1
  Product_a09bc/1 -> Add_7a2a4/1
  Constant_-1_464e4/1 -> Product_01876/1
  Product_44c38/1 -> Divide_85a6a/1
  Constant_x_l_efdef/1 -> Product_01876/2
  Product_70064/1 -> Add_9b1ee/2
  Constant_x_qd_acb58/1 -> Subtract_c083a/1
  Add_6e2e7/1 -> Product_44c38/1
  State_psi_gq_SG_D_2_84d01/1 -> Product_938d5/1
  Add_3d300/1 -> Divide_f898f/2
  Add_7a2a4/1 -> Product_938d5/2
  Product_01876/1 -> Add_1d4db/1
  Constant_x_qd_fe35b/1 -> Add_1d4db/2
  State_psi_kq_SG_D_2_c2c6b/1 -> Product_6eba8/1
  Subtract_c083a/1 -> Product_6eba8/2
  Divide_f898f/1 -> Subtract_4661a/2
  State_psi_kq_SG_D_2_8efed/1 -> Add_ca182/2
  Product_6eba8/1 -> Divide_f898f/1
  Constant_x_qdd_98767/1 -> Divide_85a6a/2
  Product_938d5/1 -> Divide_8d550/1
  Add_1d4db/1 -> Divide_8d550/2
  Constant_-1_fd960/1 -> Product_9a5e5/1
  Subtract_b77f9/1 -> Product_9a5e5/2
  Add_ca182/1 -> Subtract_56eeb/1
  Divide_85a6a/1 -> Subtract_56eeb/2
  Product_b6248/1 -> Add_78499/1
  Constant_x_qd_175a4/1 -> Add_78499/2
  Divide_8d550/1 -> Subtract_4661a/1
  Product_9a5e5/1 -> Product_d21b6/1
  Subtract_56eeb/1 -> Product_d21b6/2
  Add_78499/1 -> Power_5783a/1
  Constant_2.0_9a1e9/1 -> Power_5783a/2
  Subtract_4661a/1 -> Add_1f47e/1
  State_psi_q_SG_D_2_b4e81/1 -> Add_1f47e/2
  Product_d21b6/1 -> Divide_43dfb/1
  Power_5783a/1 -> Divide_43dfb/2
  Add_1f47e/1 -> Divide_60637/1
  Constant_x_qdd_b5603/1 -> Divide_60637/2
  Constant_x_q_fc128/1 -> Subtract_3c5b6/1
  Divide_43dfb/1 -> Subtract_6b63e/1
  Divide_60637/1 -> Subtract_6b63e/2
  Divide_58581/1 -> Blockout_d_psi_gq_SG_D_2_f38dc/1
  Constant_-1_6b382/1 -> Product_94a19/1
  State_psi_gq_SG_D_2_d4904/1 -> Product_94a19/2
  Subtract_3c5b6/1 -> Product_70064/1
  Subtract_6b63e/1 -> Product_70064/2
  Product_94a19/1 -> Add_9b1ee/1
  Add_9b1ee/1 -> Divide_58581/1
  Constant_T_qd_ddc3c/1 -> Divide_58581/2

== system case1/SG_D_2/d_psi_kq_SG_D_2_block ==
  note: d_psi_kq_SG_D_2 in case1
      | $-\frac{\psi _{\mathrm{gq},\mathrm{SG},D,2}+\psi _{\mathrm{kq},\mathrm{SG},D,2}+\frac{\left(x_{l}-x_{\mathrm{qd}}\right)\,\left(\psi _{q,\mathrm{SG},D,2}+\frac{\psi _{\mathrm{gq},\mathrm{SG},D,2}\,\left(x_{l}-x_{\mathrm{qdd}}\right)}{x_{l}-x_{\mathrm{qd}}}+\frac{\psi _{\mathrm{kq},\mathrm{SG},D,2}\,\left(x_{\mathrm{qd}}-x_{\mathrm{qdd}}\right)}{x_{l}-x_{\mathrm{qd}}}\right)}{x_{\mathrm{qdd}}}}{T_{\mathrm{qdd}}}$
      | Automatically generated on 2025-10-31 18:48:31 .
  State_psi_gq_SG_D_2_b21d1 : Inport
  State_psi_kq_SG_D_2_91d69 : Inport  Port=2
  State_psi_gq_SG_D_2_c1bff : Inport  Port=3
  State_psi_kq_SG_D_2_611bb : Inport  Port=4
  State_psi_q_SG_D_2_af7b5 : Inport  Port=5
  Add_1a62a : Sum
  Add_50783 : Sum
  Add_72eb4 : Sum
  Add_7e4b4 : Sum
  Add_e2225 : Sum
  Add_e8806 : Sum
  Constant_-1_0367a : Constant  Value=-1
  Constant_-1_1f815 : Constant  Value=-1
  Constant_-1_6bf1a : Constant  Value=-1
  Constant_-1_b37c0 : Constant  Value=-1
  Constant_-1_ec7af : Constant  Value=-1
  Constant_T_qdd_089e1 : Constant  Value=T_qdd
  Constant_x_l_4a6ab : Constant  Value=x_l
  Constant_x_l_4bcfc : Constant  Value=x_l
  Constant_x_l_8fa25 : Constant  Value=x_l
  Constant_x_l_e40e5 : Constant  Value=x_l
  Constant_x_qd_87ef2 : Constant  Value=x_qd
  Constant_x_qd_8a596 : Constant  Value=x_qd
  Constant_x_qd_97716 : Constant  Value=x_qd
  Constant_x_qd_c29e6 : Constant  Value=x_qd
  Constant_x_qdd_429d4 : Constant  Value=x_qdd
  Constant_x_qdd_ea9b8 : Constant  Value=x_qdd
  Constant_x_qdd_fdb43 : Constant  Value=x_qdd
  Divide_11400 : Product  Inputs=*/
  Divide_30da9 : Product  Inputs=*/
  Divide_3474d : Product  Inputs=*/
  Divide_92ece : Product  Inputs=*/
  Product_051d0 : Product
  Product_1465e : Product
  Product_2486d : Product
  Product_53c35 : Product
  Product_60cd9 : Product
  Product_6c7c9 : Product
  Product_8c6a3 : Product
  Product_eeb04 : Product
  Subtract_4050e : Sum  Inputs=+-
  Subtract_9dae2 : Sum  Inputs=+-
  Subtract_b21e6 : Sum  Inputs=+-
  Blockout_d_psi_kq_SG_D_2_4ff78 : Outport
  wires:
  State_psi_kq_SG_D_2_91d69/1 -> Subtract_4050e/2
  Constant_-1_1f815/1 -> Product_8c6a3/1
  Constant_-1_ec7af/1 -> Product_eeb04/1
  Constant_x_l_e40e5/1 -> Product_eeb04/2
  Constant_x_qdd_ea9b8/1 -> Add_50783/2
  Constant_x_l_8fa25/1 -> Product_8c6a3/2
  Constant_x_qd_8a596/1 -> Subtract_9dae2/1
  Constant_T_qdd_089e1/1 -> Divide_11400/2
  Constant_-1_b37c0/1 -> Product_051d0/1
  Product_eeb04/1 -> Add_50783/1
  Constant_x_qdd_fdb43/1 -> Subtract_9dae2/2
  Constant_x_l_4bcfc/1 -> Product_051d0/2
  Divide_11400/1 -> Blockout_d_psi_kq_SG_D_2_4ff78/1
  State_psi_gq_SG_D_2_c1bff/1 -> Product_1465e/1
  Add_50783/1 -> Product_1465e/2
  Product_8c6a3/1 -> Add_e8806/1
  Constant_x_qd_97716/1 -> Add_e8806/2
  Product_53c35/1 -> Divide_30da9/1
  State_psi_kq_SG_D_2_611bb/1 -> Product_60cd9/1
  Subtract_9dae2/1 -> Product_60cd9/2
  Product_051d0/1 -> Add_e2225/1
  Constant_x_qd_87ef2/1 -> Add_e2225/2
  Product_60cd9/1 -> Divide_3474d/1
  Product_1465e/1 -> Divide_92ece/1
  Add_e8806/1 -> Divide_92ece/2
  Add_e2225/1 -> Divide_3474d/2
  State_psi_q_SG_D_2_af7b5/1 -> Add_1a62a/2
  Constant_-1_6bf1a/1 -> Product_6c7c9/1
  Constant_x_l_4a6ab/1 -> Product_6c7c9/2
  Divide_92ece/1 -> Subtract_b21e6/1
  Divide_3474d/1 -> Subtract_b21e6/2
  Product_6c7c9/1 -> Add_7e4b4/1
  Constant_x_qd_c29e6/1 -> Add_7e4b4/2
  Subtract_b21e6/1 -> Add_1a62a/1
  Constant_x_qdd_429d4/1 -> Divide_30da9/2
  Constant_-1_0367a/1 -> Product_2486d/1
  State_psi_gq_SG_D_2_b21d1/1 -> Product_2486d/2
  Add_7e4b4/1 -> Product_53c35/1
  Add_1a62a/1 -> Product_53c35/2
  Product_2486d/1 -> Subtract_4050e/1
  Subtract_4050e/1 -> Add_72eb4/1
  Divide_30da9/1 -> Add_72eb4/2
  Add_72eb4/1 -> Divide_11400/1

== system case1/SG_D_2/d_psi_q_SG_D_2_block ==
  note: d_psi_q_SG_D_2 in case1
      | $2\,\pi \,f_{0}\,\left(v_{d,\mathrm{SG},D,2}\,\cos\left(\theta _{\mathrm{SG},D,2}\right)+v_{q,\mathrm{SG},D,2}\,\sin\left(\theta _{\mathrm{SG},D,2}\right)-\frac{R_{a}\,\left(\psi _{q,\mathrm{SG},D,2}+\frac{\psi _{\mathrm{gq},\mathrm{SG},D,2}\,\left(x_{l}-x_{\mathrm{qdd}}\right)}{x_{l}-x_{\mathrm{qd}}}+\frac{\psi _{\mathrm{kq},\mathrm{SG},D,2}\,\left(x_{\mathrm{qd}}-x_{\mathrm{qdd}}\right)}{x_{l}-x_{\mathrm{qd}}}\right)}{x_{\mathrm{qdd}}}-\frac{\psi _{d,\mathrm{SG},D,2}\,w_{\mathrm{SG},D,2}}{2\,f_{0}\,\pi }\right)$
      | Automatically generated on 2025-10-31 18:48:13 .
  State_psi_gq_SG_D_2_52ba9 : Inport
  State_psi_kq_SG_D_2_a91e4 : Inport  Port=2
  State_psi_q_SG_D_2_34d65 : Inport  Port=3
  Input_v_d_SG_D_2_5ea16 : Inport  Port=4
  State_theta_SG_D_2_2fc52 : Inport  Port=5
  Input_v_q_SG_D_2_1b817 : Inport  Port=6
  State_theta_SG_D_2_f1308 : Inport  Port=7
  State_psi_d_SG_D_2_1d0f8 : Inport  Port=8
  State_w_SG_D_2_df282 : Inport  Port=9
  Add_00ddb : Sum
  Add_6016b : Sum
  Add_61b86 : Sum
  Add_754da : Sum
  Add_f2b39 : Sum
  Constant_-1_38959 : Constant  Value=-1
  Constant_-1_798e0 : Constant  Value=-1
  Constant_-1_eb2e1 : Constant  Value=-1
  Constant_-2.0_fbc51 : Constant  Value=-2.0
  Constant_2.0_64429 : Constant  Value=2.0
  Constant_R_a_a6f78 : Constant  Value=R_a
  Constant_f0_18df7 : Constant  Value=f0
  Constant_f0_ac200 : Constant  Value=f0
  Constant_pi_4b7c9 : Constant  Value=pi
  Constant_pi_bede0 : Constant  Value=pi
  Constant_x_l_947aa : Constant  Value=x_l
  Constant_x_l_a6610 : Constant  Value=x_l
  Constant_x_l_cb657 : Constant  Value=x_l
  Constant_x_qd_8150e : Constant  Value=x_qd
  Constant_x_qd_95638 : Constant  Value=x_qd
  Constant_x_qd_bcaae : Constant  Value=x_qd
  Constant_x_qdd_0b8fe : Constant  Value=x_qdd
  Constant_x_qdd_693a5 : Constant  Value=x_qdd
  Constant_x_qdd_7ac7e : Constant  Value=x_qdd
  Divide_76a03 : Product  Inputs=*/
  Divide_c3130 : Product  Inputs=*/
  Divide_ed5d7 : Product  Inputs=*/
  Divide_f867b : Product  Inputs=*/
  MathFunc_cos_57b4c : Trigonometry  Operator=cos
  MathFunc_sin_354e5 : Trigonometry
  Product_4ffbc : Product
  Product_59242 : Product
  Product_6a710 : Product
  Product_76a6f : Product
  Product_7a2ea : Product
  Product_7d5bb : Product
  Product_8b076 : Product
  Product_9acaa : Product
  Product_b11d5 : Product
  Product_b47eb : Product
  Product_b71d5 : Product
  Product_d66d8 : Product
  Product_f1c65 : Product
  Product_fb970 : Product
  Subtract_1fa2e : Sum  Inputs=+-
  Subtract_79696 : Sum  Inputs=+-
  Subtract_ba3f4 : Sum  Inputs=+-
  Subtract_bedc0 : Sum  Inputs=+-
  Blockout_d_psi_q_SG_D_2_5eec6 : Outport
  wires:
  Constant_x_qdd_7ac7e/1 -> Subtract_bedc0/2
  Constant_x_l_947aa/1 -> Product_fb970/2
  Constant_-1_eb2e1/1 -> Product_4ffbc/1
  Constant_x_l_a6610/1 -> Product_4ffbc/2
  Product_4ffbc/1 -> Add_61b86/1
  Constant_pi_4b7c9/1 -> Product_8b076/2
  State_psi_gq_SG_D_2_52ba9/1 -> Product_b47eb/1
  Constant_x_l_cb657/1 -> Product_59242/2
  State_w_SG_D_2_df282/1 -> Product_6a710/2
  Constant_x_qd_bcaae/1 -> Add_f2b39/2
  Constant_x_qdd_693a5/1 -> Add_61b86/2
  Constant_2.0_64429/1 -> Product_8b076/1
  Constant_-1_798e0/1 -> Product_59242/1
  Constant_x_qd_95638/1 -> Subtract_bedc0/1
  Constant_-1_38959/1 -> Product_fb970/1
  State_psi_q_SG_D_2_34d65/1 -> Add_754da/2
  Add_61b86/1 -> Product_b47eb/2
  Product_8b076/1 -> Product_76a6f/1
  Product_59242/1 -> Add_00ddb/1
  Constant_pi_bede0/1 -> Product_d66d8/2
  Constant_f0_18df7/1 -> Product_76a6f/2
  Constant_x_qd_8150e/1 -> Add_00ddb/2
  State_psi_kq_SG_D_2_a91e4/1 -> Product_b11d5/1
  Subtract_bedc0/1 -> Product_b11d5/2
  Product_fb970/1 -> Add_f2b39/1
  Input_v_q_SG_D_2_1b817/1 -> Product_7d5bb/1
  Product_b47eb/1 -> Divide_ed5d7/1
  Product_76a6f/1 -> Divide_f867b/2
  Add_00ddb/1 -> Divide_ed5d7/2
  Product_b11d5/1 -> Divide_c3130/1
  Add_f2b39/1 -> Divide_c3130/2
  Divide_ed5d7/1 -> Subtract_1fa2e/1
  State_theta_SG_D_2_2fc52/1 -> MathFunc_cos_57b4c/1
  Divide_c3130/1 -> Subtract_1fa2e/2
  Subtract_1fa2e/1 -> Add_754da/1
  MathFunc_cos_57b4c/1 -> Product_7a2ea/2
  Constant_R_a_a6f78/1 -> Product_b71d5/1
  Add_754da/1 -> Product_b71d5/2
  State_theta_SG_D_2_f1308/1 -> MathFunc_sin_354e5/1
  Product_b71d5/1 -> Divide_76a03/1
  Product_d66d8/1 -> Product_9acaa/1
  Product_7d5bb/1 -> Subtract_79696/2
  Constant_x_qdd_0b8fe/1 -> Divide_76a03/2
  Input_v_d_SG_D_2_5ea16/1 -> Product_7a2ea/1
  Add_6016b/1 -> Product_f1c65/2
  Divide_76a03/1 -> Subtract_ba3f4/1
  Product_7a2ea/1 -> Subtract_ba3f4/2
  MathFunc_sin_354e5/1 -> Product_7d5bb/2
  Product_f1c65/1 -> Blockout_d_psi_q_SG_D_2_5eec6/1
  State_psi_d_SG_D_2_1d0f8/1 -> Product_6a710/1
  Constant_-2.0_fbc51/1 -> Product_d66d8/1
  Product_9acaa/1 -> Product_f1c65/1
  Subtract_ba3f4/1 -> Subtract_79696/1
  Product_6a710/1 -> Divide_f867b/1
  Constant_f0_ac200/1 -> Product_9acaa/2
  Subtract_79696/1 -> Add_6016b/1
  Divide_f867b/1 -> Add_6016b/2

== system case1/SG_D_2/d_theta_SG_D_2_block ==
  note: d_theta_SG_D_2 in case1
      | $w_{\mathrm{SG},D,2}-2\,\pi \,f_{0}$
      | Automatically generated on 2025-10-31 18:48:39 .
  State_w_SG_D_2_5c0a1 : Inport
  Add_102e3 : Sum
  Constant_-2.0_3901b : Constant  Value=-2.0
  Constant_f0_f3d5e : Constant  Value=f0
  Constant_pi_2a675 : Constant  Value=pi
  Product_05e14 : Product
  Product_dff6c : Product
  Blockout_d_theta_SG_D_2_6c47c : Outport
  wires:
  Constant_-2.0_3901b/1 -> Product_dff6c/1
  Constant_pi_2a675/1 -> Product_dff6c/2
  Add_102e3/1 -> Blockout_d_theta_SG_D_2_6c47c/1
  Product_dff6c/1 -> Product_05e14/1
  Constant_f0_f3d5e/1 -> Product_05e14/2
  Product_05e14/1 -> Add_102e3/1
  State_w_SG_D_2_5c0a1/1 -> Add_102e3/2
